simulink model "psk"  (Simulink 9.3)
settings: Solver=VariableStepAuto  StartTime=0.0  StopTime=1/15  RelTol=1e-3
undefined symbols (not defined in the file or in its folder): gray
libraries: commutil2 x2, commdigbbndpm3 x2, commchan3 x1, commsink2 x1, visionsources x1
settings Model: Creator=triud  LastModifiedBy=triud
settings DataIOCC: SaveFormat=Dataset  SignalLoggingSaveFormat=Dataset  ReturnWorkspaceOutputs=on
settings OptimizationCC: LifeSpan=auto
settings DebuggingCC: UnderspecifiedInitializationDetection=Simplified  MergeDetectMultiDrivingBlocksExec=error  FcnCallInpInsideContextMsg=error  SFUnexpectedBacktrackingDiag=error  SFNoUnconditionalDefaultTransitionDiag=error  SFExecutionAtInitializationDiag=warning  ArithmeticOperatorsInVariantConditions=error
settings HardwareCC: ProdBitPerPointer=64  ProdBitPerSizeT=64  ProdBitPerPtrDiffT=64  ProdLargestAtomicFloat=Float  ProdIntDivRoundTo=Zero  ProdEndianess=LittleEndian  ProdWordSize=64  ProdHWDeviceType=Intel->x86-64 (Windows64)
settings ModelReferenceCC: PropagateSignalLabelsOutOfModel=on
settings SFSimCC: SimUseLocalCustomCode=on
settings RTWCC: RTWUseLocalCustomCode=on
settings CodeAppCC: StateflowObjectComments=off
settings GRTTargetCC: TargetLangStandard=C99 (ISO)  CombineOutputUpdateFcns=on  GRTInterface=off
settings ConfigComp: CovMetricSettings=dwe  CovHtmlReporting=off  CovSaveCumulativeToWorkspaceVar=off  CovSaveSingleToWorkspaceVar=off  CovExternalEMLEnable=on

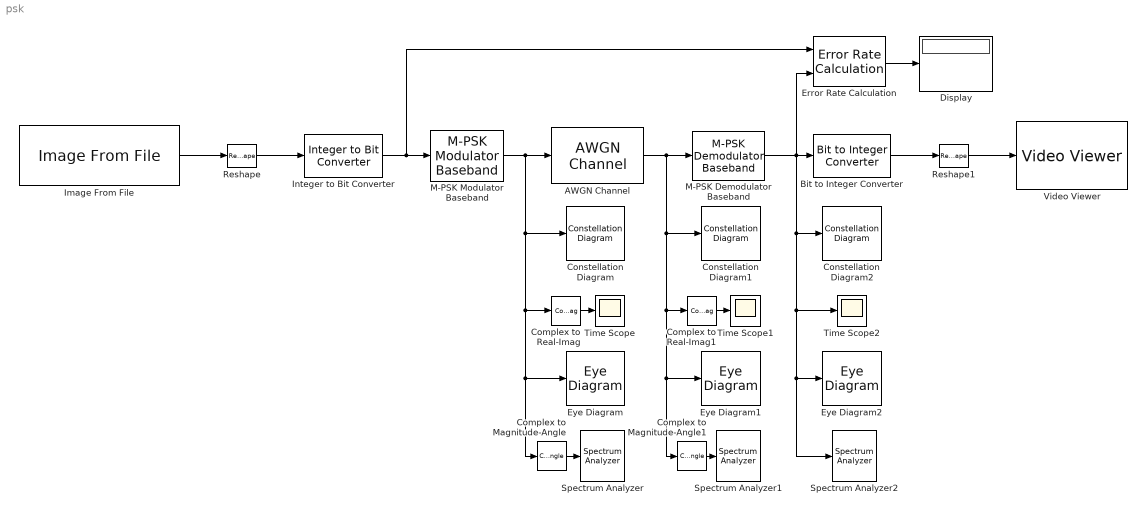
== system psk ==
  AWGN Channel : commchan3/AWGN Channel  InputProcessing=Columns as channels (frame based)  seed=67  noiseMode="Signal to noise ratio  (SNR)"  EbNodB=10  EsNodB=10  SNRdB=5  bitsPerSym=1  Ps=1  Tsym=1  variance=1
      settings: SourceProductName=Communications Toolbox
  Bit to Integer Converter : commutil2/Bit to Integer Converter  nbits=8  bitOrder=LSB first  signedOutputValues=Unsigned  outDtype=Inherit via internal rule  outDtypeSigned=Inherit via internal rule
      settings: SourceProductName=Communications Toolbox
  Complex to Magnitude-Angle : ComplexToMagnitudeAngle  Output=Magnitude
  Complex to Magnitude-Angle1 : ComplexToMagnitudeAngle  Output=Magnitude
  Complex to Real-Imag : ComplexToRealImag  Output=Real
  Complex to Real-Imag1 : ComplexToRealImag  Output=Real
  Constellation Diagram : ConstellationDiagram
  Constellation Diagram1 : ConstellationDiagram
  Constellation Diagram2 : ConstellationDiagram
  Display : Display
  Error Rate Calculation : commsink2/Error Rate Calculation  N=0  st_delay=0  cp_mode=Entire frame  subframe=[]  PMode=Port  WsName=ErrorVec  RsMode2=off  stop=off  numErr=100  maxBits=1e6
      settings: SourceProductName=Communications Toolbox
  Eye Diagram : EyeDiagram
  Eye Diagram1 : EyeDiagram
  Eye Diagram2 : EyeDiagram
  Image From File : visionsources/Image From File  Tag=vipblks_nd  FileName=D:\matlab\workspace\btl\y2025VinhHaLong.jpeg  Ts=1/15  imagePorts=One multidimensional signal  OutPortLabels=R|G|B  ImageDataType=Inherit from input image  sdImageDataType=uint(8)  Signed=on  WordLength=16  FractionLengthMode=User-defined  FractionLength=15
      settings: SourceProductName=Computer Vision Toolbox
  Integer to Bit Converter : commutil2/Integer to Bit Converter  nbits=8  signedInputValues=Unsigned  bitOrder=LSB first  outDtype=Inherit via internal rule
      settings: SourceProductName=Communications Toolbox
  M-PSK Demodulator Baseband : commdigbbndpm3/M-PSK Demodulator Baseband  M=64  OutType=Bit  DecType=Hard decision  VarSource=Dialog  Variance=1  Dec=Gray  Mapping=[0:7]  Ph=pi/8  outDtype1=uint8  outDtype2=Inherit via internal rule  derotateFactorWordLen=16  derotateFactorDataTypeStr=Inherit: Same word length as input  derotateFactorLastDataTypeStr=Inherit: Same word length as input
      settings: SourceProductName=Communications Toolbox
  M-PSK Modulator Baseband : commdigbbndpm3/M-PSK Modulator Baseband  M=64  InType=Bit  Enc=Gray  Mapping=[0:7]  Ph=pi/8  outDtype=double  outWordLen=16  outUDDataType=sfix(16)  outFracLenMode=Best precision  outFracLen=15  outDataTypeStr=double  outLastDataTypeStr=double
      settings: SourceProductName=Communications Toolbox
  Reshape : Reshape
  Reshape1 : Reshape  OutputDimensionality=Customize  OutputDimensions=[354,660,3]
  Spectrum Analyzer : SpectrumAnalyzer
  Spectrum Analyzer1 : SpectrumAnalyzer
  Spectrum Analyzer2 : SpectrumAnalyzer
  Time Scope : Scope
  Time Scope1 : Scope
  Time Scope2 : Scope
  Video Viewer : VideoViewer  colormapValue=gray(256)  FigPos=[1 670 1280 570]
  wires:
  Image From File/1 -> Reshape/1
  Reshape/1 -> Integer to Bit Converter/1
  Integer to Bit Converter/1 -> M-PSK Modulator Baseband/1, Error Rate Calculation/1
  M-PSK Modulator Baseband/1 -> Complex to Magnitude-Angle/1, Eye Diagram/1, Complex to Real-Imag/1, Constellation Diagram/1, AWGN Channel/1
  Bit to Integer Converter/1 -> Reshape1/1
  Reshape1/1 -> Video Viewer/1
  Error Rate Calculation/1 -> Display/1
  Complex to Real-Imag/1 -> Time Scope/1
  Complex to Magnitude-Angle/1 -> Spectrum Analyzer/1
  Complex to Real-Imag1/1 -> Time Scope1/1
  Complex to Magnitude-Angle1/1 -> Spectrum Analyzer1/1
  AWGN Channel/1 -> M-PSK Demodulator Baseband/1, Constellation Diagram1/1, Complex to Real-Imag1/1, Eye Diagram1/1, Complex to Magnitude-Angle1/1
  M-PSK Demodulator Baseband/1 -> Error Rate Calculation/2, Bit to Integer Converter/1, Time Scope2/1, Spectrum Analyzer2/1, Eye Diagram2/1, Constellation Diagram2/1
